simulink model "feedback_zd"  (R2022b)
settings: Solver=VariableStepAuto  StartTime=0.0  StopTime=10.0  RelTol=10-6
model workspace (MAT data in the model file):
  kd1 = Simulink.Parameter
  kd1.Value = 2
  kd1.DataType = 'auto'
  kd1.Complexity = 'real'
  kd1.Dimensions = [1 1]
  kd2 = Simulink.Parameter
  kd2.Value = 2
  kd2.DataType = 'auto'
  kd2.Complexity = 'real'
  kd2.Dimensions = [1 1]
  kp1 = Simulink.Parameter
  kp1.Value = 2
  kp1.DataType = 'auto'
  kp1.Complexity = 'real'
  kp1.Dimensions = [1 1]
  kp2 = Simulink.Parameter
  kp2.Value = 2
  kp2.DataType = 'auto'
  kp2.Complexity = 'real'
  kp2.Dimensions = [1 1]
libraries: robotmobilelib x1
settings Model: Creator=thoma  LastModifiedBy=borgh
settings DebuggingCC: AlgebraicLoopMsg=none  UnderSpecifiedDimensionMsg=warning

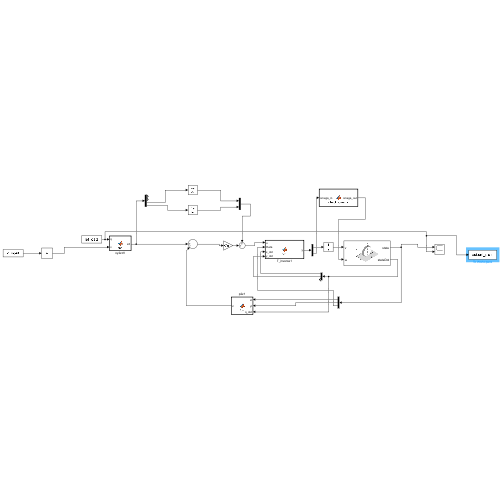
[thumbnail: Simulink's stored preview of the top-level diagram]
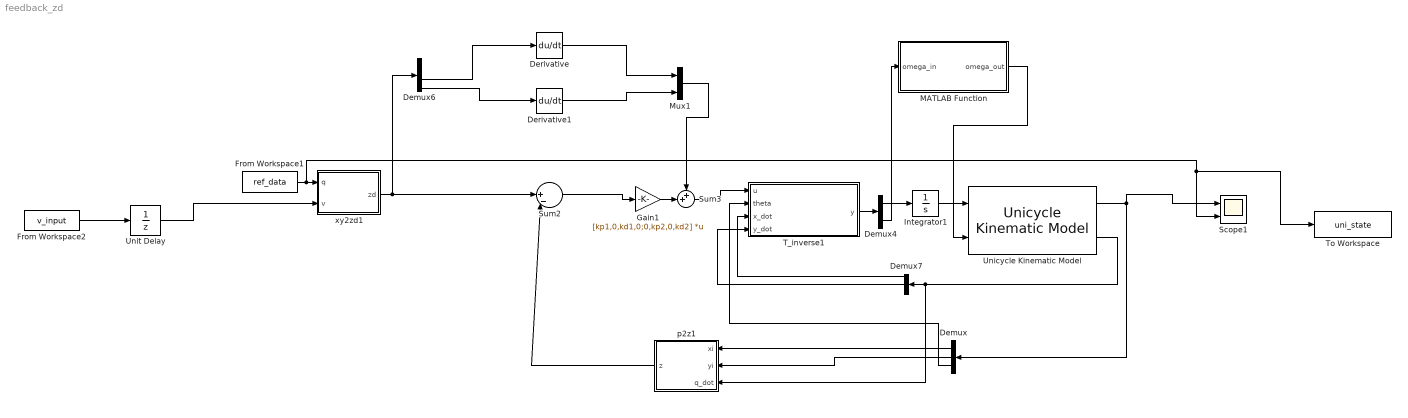
== system feedback_zd ==
  Demux : Demux  Outputs=3
  Demux4 : Demux  Outputs=2
  Demux6 : Demux
  Demux7 : Demux  Outputs=3
  Derivative : Derivative
  Derivative1 : Derivative
  From Workspace1 : FromWorkspace  VariableName=ref_data
  From Workspace2 : FromWorkspace  VariableName=v_input
  Gain1 : Gain  Gain=[kp1,0,kd1,0;0,kp2,0,kd2]  Multiplication=Matrix(K*u)
  Integrator1 : Integrator
  MATLAB Function : MATLAB Function  TreatAsAtomicUnit=on
  Mux1 : Mux  Inputs=2
  Scope1 : Scope  NumInputPorts=2
  Sum2 : Sum  Inputs=||+-|
  Sum3 : Sum  Inputs=++|
  T_inverse1 : MATLAB Function  TreatAsAtomicUnit=on
  To Workspace : ToWorkspace  VariableName=uni_state  SaveFormat=Structure With Time  SampleTime=0.1
  Unicycle Kinematic Model : robotmobilelib/Unicycle Kinematic Model  VehicleInputs=Vehicle Speed & Heading Angular Velocity  WheelRadius=2  WheelSpeedRange=[-Inf Inf]  InitialState=[125; 60; 0]  SimulateUsing=Interpreted execution
  Unit Delay : UnitDelay  SampleTime=-1  HasFrameUpgradeWarning=on
  p2z1 : MATLAB Function  TreatAsAtomicUnit=on
  xy2zd1 : MATLAB Function  TreatAsAtomicUnit=on
  wires:
  From Workspace1/1 -> To Workspace/1, Scope1/2, xy2zd1/1(q)
  T_inverse1/1(y) -> Demux4/1
  Gain1/1 -> Sum3/2
  Demux4/1 -> Integrator1/1
  Sum3/1 -> T_inverse1/1(u)
  xy2zd1/1(zd) -> Sum2/1, Demux6/1
  Mux1/1 -> Sum3/1
  p2z1/1(z) -> Sum2/2
  Unicycle Kinematic Model/1 -> Scope1/1, Demux/1
  Integrator1/1 -> Unicycle Kinematic Model/1
  Unicycle Kinematic Model/2 -> p2z1/3(q_dot), Demux7/1
  Demux7/1 -> T_inverse1/3(x_dot)
  Demux7/2 -> T_inverse1/4(y_dot)
  Demux/1 -> p2z1/1(xi)
  Demux/2 -> p2z1/2(yi)
  Demux6/3 -> Derivative/1
  Derivative/1 -> Mux1/1
  Derivative1/1 -> Mux1/2
  Demux4/2 -> MATLAB Function/1(omega_in)
  MATLAB Function/1(omega_out) -> Unicycle Kinematic Model/2
  Sum2/1 -> Gain1/1
  Demux/3 -> T_inverse1/2(theta)
  Demux6/4 -> Derivative1/1
  From Workspace2/1 -> Unit Delay/1
  Unit Delay/1 -> xy2zd1/2(v)

== matlab function feedback_zd/MATLAB Function ==
  data: omega_in input; omega_out output
function omega_out = check_omega(omega_in)
    % Check if omega (angular velocity) is finite
    if ~isfinite(omega_in)
        omega_out = 0;  % Set omega to a default value, e.g., 0 if it is NaN or Inf
    else
        omega_out = omega_in;  % Otherwise, pass the input value
    end
end

== matlab function feedback_zd/T_inverse1 ==
  data: u input; y output; theta input; x_dot input; y_dot input
function y = fcn(u,theta,x_dot,y_dot)
v=sqrt(x_dot^2+y_dot^2);
theta=mod(theta+pi,2*pi)-pi;
T_inverse=[cos(theta),sin(theta);-sin(theta)/v,cos(theta)/v];
vet=T_inverse*u;
y = vet;

== matlab function feedback_zd/p2z1 ==
  data: xi input; yi input; z output; q_dot input
function z = fcn(xi,yi, q_dot)
x_dot = q_dot(1);
y_dot = q_dot(2);
z = [xi; yi; x_dot; y_dot];  % z is a 4x1 vecto

== matlab function feedback_zd/xy2zd1 ==
  data: q input; zd output; v input
function zd = fcn(q,v)
x=q(1);
y=q(2);
theta=q(3);
theta=mod(theta+pi,2*pi)-pi;
z3=v*cos(theta);
z4=v*sin(theta);
zd=[x;y;z3;z4];
